simulink model "TransferFunction"  (R2023a)
settings: Solver=VariableStepAuto  StartTime=0.0  StopTime=10.0  RelTol=1e-3
settings Model: Creator=NG22  LastModifiedBy=NG22

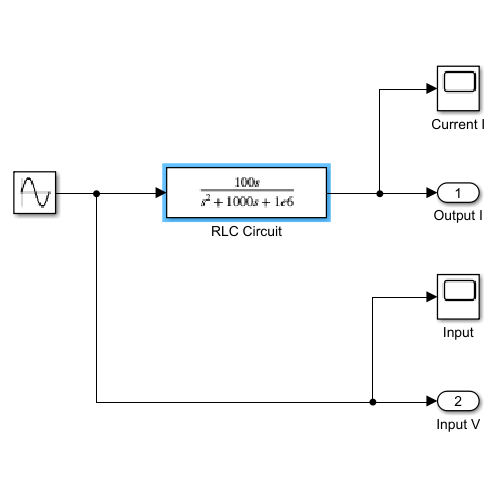
[thumbnail: Simulink's stored preview of the top-level diagram]
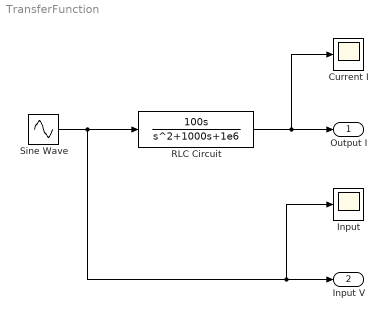
== system TransferFunction ==
  Current I : Scope
  Input : Scope
  RLC Circuit : TransferFcn  Numerator=[100 0]  Denominator=[1 1000 1e6]
  Sine Wave : Sin  SampleTime=0
  Output I : Outport
  Input V : Outport  Port=2
  wires:
  RLC Circuit/1 -> Current I/1, Output I/1
  Sine Wave/1 -> RLC Circuit/1, Input/1, Input V/1
